simulink model "MultirotorSimPx4"  (R2018b)
settings: Solver=VariableStepAuto  StartTime=0.0  StopTime=Simulation.T_END  MaxStep=Simulation.TS_MAX  RelTol=1e-3  EnableMultiTasking=on
PreLoadFcn:
  | % InitializeParameters;
undefined symbols (not defined in the file): Aero, Initial, Motor, Simulation, Uav
libraries: QuaternionLibrary x13, simulink_extras x9, Px4Library x4, simulink x1
(part 3 of 8)

== matlab function MultirotorSimPx4/Quadrotor Quaternion Model/Equations of motion ==
  data: VBody input; VBodyDot output; nuBody input; Q input; TBody input size=3; tauBody input size=3; F_D input size=3; M_D input size=3; time input; nuBodyDot output; Uav parameter; xiDDot output; Simulation parameter
function [VBodyDot, nuBodyDot, xiDDot] = QuadrotorQuaternionModel(...
    VBody, nuBody, Q, TBody, tauBody, F_D, M_D, time, Uav, Simulation)
%#codegen

%% Handle 2D pitch test
if isfield( Uav, 'PITCH_ONLY') && Uav.PITCH_ONLY
    tauBody = [0; 1; 0] .* tauBody;
    M_D = [0; 1; 0] .* M_D;
end

if isfield( Simulation, 'T_START_STEP') && ( time < Simulation.T_START_STEP )
    tauBody = [0; 0; 0] .* tauBody;
    M_D = [0; 0; 0] .* M_D;
end

%% Moments and Forces
% Body frame accelerations
VBodyDot  = (1/Uav.M) * (Q'*Uav.G + TBody - cross(nuBody, Uav.M*VBody) + F_D);
nuBodyDot = Uav.I \ (tauBody - cross(nuBody, Uav.I*nuBody) + M_D);

% Inertial frame accelerations
xiDDot = (1/Uav.M)*(Uav.G + Q*(TBody + F_D));
% etaDDot = WInvertDot*nuBody + WInvert*nuBodyDot;

% Check centripetal force in inertial frame
% F_C = R*cross(nuBody,m*VBody);

if Uav.PITCH_ONLY
    xiDDot = [1; 1; 0] .* xiDDot;
end

end

== matlab function MultirotorSimPx4/Compute Sph ==
  data: V_appBody input; azimuth output; elevation output; radius output
function [azimuth, elevation, radius] = computeSph(V_appBody)
%#codegen

% Convert from polar to spherical coordinates
[ azimuth, elevation, radius ] = cart2sph( V_appBody(1), V_appBody(2), V_appBody(3) );

== matlab function MultirotorSimPx4/att_controller_ff ==
  data: Textra input; thrustDes output [0..1]; V_appBody input size=3; q input; omega input; Motor parameter; Uav parameter; Aero parameter
function thrustDes  = ffThrust( Textra, V_appBody, q, omega, Motor, Uav, Aero )
%#codegen
    [ azimuth, elevation, windSpeed ] = cart2sph( V_appBody(1), V_appBody(2), V_appBody(3) );
    
    R = QuatToRot(q);
    Rz = R(:,3);
    vertical = [0; 0; 1];
    
    alpha = atan2( norm(cross( Rz, vertical )), dot( Rz, vertical ) );

    if strcmp( Aero.Type, 'Body oriented' )
        U = windSpeed;
        lambda = mean(omega .* Uav.D_PROP / ( 2 * U ));
        
        Cz1 = dot( Aero.Cz1.coefs, [sin(alpha), 1] );
        fz_lift = 0.5 .* Uav.RHO_AIR .* U^2 .* Cz1 * Uav.A_UAV;

        Cz2 = dot( Aero.Cz2.coefs, [alpha, 1]);
        p = Aero.Cz3.coefs;
        Cz3 = p(1) * sin(alpha) + p(2) * ( 1 - exp(-p(3).*lambda) ) .* sin(3*alpha) + ...
            p(4);
        a = 0.5 .* Uav.RHO_AIR .* Cz2 .* Uav.D_PROP^2 .* Uav.A_PROP; % Rotor thrust
        b = 0.5 .* Uav.RHO_AIR .* Cz3 .* U .* Uav.D_PROP .* Uav.A_PROP; % Rotor thrust correction
        
        mg = Uav.G(3);
        Trequired = ((mg / cos(alpha)) - (fz_lift) + Textra)/Uav.N_ROTORS;
        c = Trequired;
        
        omegaRefDes = (-b + sqrt(b^2 + 4*a*c) )/(2*a);
    else
        % Thrust
        x1 = sin(-elevation);
        x2 = windSpeed;
        CT1 = 0.5 * Uav.RHO_AIR * dot( Aero.CT1.coefs, [ 1, x1, x2, x1*x2, x1^2, x2^2, x1^2*x2^2  ] );
        CT2 = 0.5 * Uav.RHO_AIR * dot( Aero.CT2.coefs, [ 1, x1, x2, x1*x2, x1^2, x2^2, x1^2*x2^2  ] );

        % Drag
        x1 = cos(-elevation);
        x2 = mean(omega);
        Cd1 = dot( Aero.Cd1.coefs, [ 1, x1, x2, x1*x2, x1^2, x2^2, x1^2*x2^2  ] );
        Cd2 = dot( Aero.Cd2.coefs, [ 1, x1, x2, x1*x2, x1^2, x2^2, x1^2*x2^2  ] );
        f_D = 0.5 * Uav.RHO_AIR * Cd1 * windSpeed^2 + ...
        0.5 * Uav.RHO_AIR * Cd2 * windSpeed;

        % Lift
        x1 = -elevation;
        x2 = 0;
        Cl = dot( Aero.Cl.coefs, [ 1, x1, x2, x1*x2, x1^2, x2^2, x1^2*x2^2  ] );
        f_l = 0.5 * Uav.RHO_AIR * Cl * windSpeed^2;

        F_D = zeros(3,1);
        F_l = zeros(3,1);
        [ F_D(1), F_D(2), F_D(3) ] = sph2cart( azimuth, elevation, f_D );
        [ F_l(1), F_l(2), F_l(3) ] = sph2cart( azimuth, elevation + pi/2, f_l );

        mg = -Uav.G(3);
        Trequired = mg / cos(alpha) - (F_l(3) + F_D(3)) + Textra;

        omegaRefDes = (-CT2 + sqrt(CT2^2 + 4*CT1*Trequired) )/(2*CT1);
    end


    omegaDes = omegaRefDes; %- mean(omegaDot)*7.006512e-02;
    pwmDes = ( omegaDes/0.84 + 6.528579e2) / 7.969173e-1;

    thrustDes = (pwmDes - 1000) / 1000;
end

function R = QuatToRot( q )
% QUATERNIONTOROTATIONMATRIXMAT Convert quaternion to rotation matrix
% Written by: J.X.J. Bannwarth, 27/03/17
    W = q(1);
    X = q(2);
    Y = q(3);
    Z = q(4);
    
    xx = X * X;
    xy = X * Y;
    xz = X * Z;
    xw = X * W;

    yy = Y * Y;
    yz = Y * Z;
    yw = Y * W;
    
    zz = Z * Z;
    zw = Z * W;

    m00 = 1 - 2 * ( yy + zz );
    m01 =     2 * ( xy - zw );
    m02 =     2 * ( xz + yw );

    m10 =     2 * ( xy + zw );
    m11 = 1 - 2 * ( xx + zz );
    m12 =     2 * ( yz - xw );

    m20 =     2 * ( xz - yw );
    m21 =     2 * ( yz + xw );
    m22 = 1 - 2 * ( xx + yy );
    
    R = [m00 m01 m02;
         m10 m11 m12;
         m20 m21 m22];
    
end

== matlab function MultirotorSimPx4/Applied wind speed/Relative velocity ==
  data: nuBody input; Uav parameter; VMotorRelBody output
function VMotorRelBody = relativeMotorVelocity( nuBody , Uav )
%#codegen
    VMotorRelBody = cross( nuBody, Uav.L_VEC );
end

== matlab function MultirotorSimPx4/Applied wind speed/Compute V_app2 ==
  data: Q input; UBody output; U input size=3
function UBody = computeUBody(Q, U)
%#codegen

% Rotation matrix from Wind frame to Inertial frame
% Wind frame SEU, inertial frame NED
R_U = [1,  0, 0;
       0, -1, 0;
       0,  0, 1];
   
UBody = Q' * R_U * U;

== matlab function MultirotorSimPx4/att_mixerInput/Euler Angles to Quaternion/MATLAB Function ==
  data: eulerAngles input; quat output
function quat   = EulerToQuaternion( eulerAngles )
%EULERTOQUATERNION Convert Euler angles to a quaternion
%   Based on PX4 Firmware code: https://github.com/PX4/Firmware
%   Written by: J.X.J. Bannwarth
%   Last modified: 29/08/2016

    roll  = eulerAngles(1);
    pitch = eulerAngles(2);
    yaw   = eulerAngles(3);

    cosPhi_2   = cos(roll / 2.0);
    sinPhi_2   = sin(roll / 2.0);
    cosTheta_2 = cos(pitch / 2.0);
    sinTheta_2 = sin(pitch / 2.0);
    cosPsi_2   = cos(yaw / 2.0);
    sinPsi_2   = sin(yaw / 2.0);

    quat = [ cosPhi_2 .* cosTheta_2 .* cosPsi_2 + sinPhi_2 .* sinTheta_2 .* sinPsi_2;
             sinPhi_2 .* cosTheta_2 .* cosPsi_2 - cosPhi_2 .* sinTheta_2 .* sinPsi_2;
             cosPhi_2 .* sinTheta_2 .* cosPsi_2 + sinPhi_2 .* cosTheta_2 .* sinPsi_2;
             cosPhi_2 .* cosTheta_2 .* sinPsi_2 - sinPhi_2 .* sinTheta_2 .* cosPsi_2 ];

end

== matlab function MultirotorSimPx4/Sensor Model/Global reprojection/map_projection_reproject ==
  data: x input; y input; lat output; lon output; LAT0 parameter; LON0 parameter
function [ lat, lon ] = map_projection_reproject( x, y, LAT0, LON0)
%#codegen
%MAP_PROJECTION_REPROJECT
    M_DEG_TO_RAD = 0.017453292519943295;
	ref.lat_rad = LAT0 * M_DEG_TO_RAD;
	ref.lon_rad = LON0 * M_DEG_TO_RAD;
	ref.sin_lat = 0;
	ref.cos_lat = 0; 
    ref.sin_lat = sin(ref.lat_rad);
    ref.cos_lat = cos(ref.lat_rad);
    
    CONSTANTS_RADIUS_OF_EARTH = 6371000;
    M_PI = 3.14159265358979323846;

    x_rad = x / CONSTANTS_RADIUS_OF_EARTH;
    y_rad = y / CONSTANTS_RADIUS_OF_EARTH;
    c = sqrt(x_rad * x_rad + y_rad * y_rad);
    
    sin_c = sin(c);
    cos_c = cos(c);

    if (abs(c) > eps)
        lat_rad = asin(cos_c * ref.sin_lat + (x_rad * sin_c * ref.cos_lat) / c);
        lon_rad = (ref.lon_rad + atan2(y_rad * sin_c, c * ref.cos_lat * cos_c - x_rad * ref.sin_lat * sin_c));
    else
        lat_rad = ref.lat_rad;
        lon_rad = ref.lon_rad;
    end

    lat = lat_rad * 180.0 / M_PI;
    lon = lon_rad * 180.0 / M_PI;
end

== matlab function MultirotorSimPx4/att_mixerInput/Quaternion to Euler Angles3/MATLAB Function ==
  data: quat input; eul output
function eul   = QuaternionToEuler( quat )
%QUATERNIONTOEULER Convert quaternion to euler angles
%   Based on PX4 Firmware code: https://github.com/PX4/Firmware
%   Written by:    J.X.J. Bannwarth, 2016/08/29
%   Last modified: J.X.J. Bannwarth, 2018/12/11

    eul = [ atan2(2.0 .* (quat(1) .* quat(2) + quat(3) .* quat(4)), ...
                1.0 - 2.0 .* (quat(2) .* quat(2) + quat(3) .* quat(3)));
	        asin(2.0 .* (quat(1) .* quat(3) - quat(4) .* quat(2)));
            atan2(2.0 .* (quat(1) .* quat(4) + quat(2) .* quat(3)), ...
                1.0 - 2.0 .* (quat(3) .* quat(3) + quat(4) .* quat(4))) ];
end

== matlab function MultirotorSimPx4/Sensor Model/attitude_estimator_q/Input assignment q ==
  data: airspeed_sub_indicated_airspeed_m_s input; airspeed_sub_timestamp input; global_pos_sub_eph input; global_pos_sub_lat input; global_pos_sub_lon input; global_pos_sub_timestamp input; global_pos_sub_vel_n input; global_pos_sub_vel_e input; global_pos_sub_vel_d input; mocap_sub_q input; mocap_sub_timestamp input; sensors_sub_timestamp input; sensors_sub_gyro_rad input; sensors_sub_accelerometer_m_s2 input; sensors_sub_accelerometer_timestamp_relative input; sensors_sub_magnetometer_ga input; sensors_sub_magnetometer_timestamp_relative input; selfVecIn input; selfVec output
function selfVec = InputAssignment( ...
	     airspeed_sub_indicated_airspeed_m_s, ...
	                  airspeed_sub_timestamp, ...
	                      global_pos_sub_eph, ...
	                      global_pos_sub_lat, ...
	                      global_pos_sub_lon, ...
	                global_pos_sub_timestamp, ...
	                    global_pos_sub_vel_n, ...
	                    global_pos_sub_vel_e, ...
	                    global_pos_sub_vel_d, ...
	                             mocap_sub_q, ...
	                     mocap_sub_timestamp, ...
	                   sensors_sub_timestamp, ...
	                    sensors_sub_gyro_rad, ...
	          sensors_sub_accelerometer_m_s2, ...
	sensors_sub_accelerometer_timestamp_relative, ...
	             sensors_sub_magnetometer_ga, ...
	sensors_sub_magnetometer_timestamp_relative, ...
	                               selfVecIn ...
	)
%#codegen

	selfVec = selfVecIn;

	% Variable assignment
	selfVec(10:10) =      airspeed_sub_indicated_airspeed_m_s;
	selfVec(11:11) =                   airspeed_sub_timestamp;
	selfVec(45:45) =                       global_pos_sub_eph;
	selfVec(46:46) =                       global_pos_sub_lat;
	selfVec(47:47) =                       global_pos_sub_lon;
	selfVec(48:48) =                 global_pos_sub_timestamp;
	selfVec(50:50) =                     global_pos_sub_vel_n;
	selfVec(51:51) =                     global_pos_sub_vel_e;
	selfVec(52:52) =                     global_pos_sub_vel_d;
	selfVec(147:150) =                              mocap_sub_q;
	selfVec(151:151) =                      mocap_sub_timestamp;
	selfVec(166:166) =                    sensors_sub_timestamp;
	selfVec(168:170) =                     sensors_sub_gyro_rad;
	selfVec(171:173) =           sensors_sub_accelerometer_m_s2;
	selfVec(174:174) = sensors_sub_accelerometer_timestamp_relative;
	selfVec(175:177) =              sensors_sub_magnetometer_ga;
	selfVec(178:178) = sensors_sub_magnetometer_timestamp_relative;
end

== matlab function MultirotorSimPx4/Sensor Model/attitude_estimator_q/Output selection q ==
  data: att_pub_timestamp output; att_pub_rollspeed output; att_pub_pitchspeed output; att_pub_yawspeed output; att_pub_q output; selfVec input; ctrl_state_pub_x_acc output; ctrl_state_pub_y_acc output; ctrl_state_pub_z_acc output
function [ ...
                        att_pub_timestamp, ...
                        att_pub_rollspeed, ...
                       att_pub_pitchspeed, ...
                         att_pub_yawspeed, ...
                                att_pub_q, ...
                     ctrl_state_pub_x_acc, ...
                     ctrl_state_pub_y_acc, ...
                     ctrl_state_pub_z_acc] ...
   = OutputSelection( selfVec )
%#codegen

	% Variable assignment
	                       att_pub_timestamp = selfVec(14:14);
	                       att_pub_rollspeed = selfVec(15:15);
	                      att_pub_pitchspeed = selfVec(16:16);
	                        att_pub_yawspeed = selfVec(17:17);
	                               att_pub_q = selfVec(18:21);
	                    ctrl_state_pub_x_acc = selfVec(29:29);
	                    ctrl_state_pub_y_acc = selfVec(30:30);
	                    ctrl_state_pub_z_acc = selfVec(31:31);
end
